simulink model "vllms_4_tap"  (R2021a)
settings: Solver=VariableStepDiscrete  StartTime=0.0  StopTime=4000  MaxStep=1.0  RelTol=1e-3  EnableMultiTasking=on
libraries: dspsrcs4 x2
settings Model: Creator=HP  LastModifiedBy=HP
settings SolverCC: AlgebraicLoopSolver=TrustRegion
settings DataIOCC: ReturnWorkspaceOutputs=off
settings OptimizationCC: LifeSpan=inf
settings DebuggingCC: SFUnexpectedBacktrackingDiag=warning  SFNoUnconditionalDefaultTransitionDiag=warning  SFMachineParentedDataDiag=warning  ArithmeticOperatorsInVariantConditions=warning
settings SFSimCC: SimUseLocalCustomCode=off  CustomCodeUndefinedFunction=UseInterfaceOnly
settings RTWCC: RTWUseLocalCustomCode=off
settings CodeAppCC: StateflowObjectComments=on
settings GRTTargetCC: TargetLangStandard=C89/C90 (ANSI)
settings ConfigComp: CovMetricSettings=dw  CovSaveCumulativeToWorkspaceVar=on  CovSaveSingleToWorkspaceVar=on  CovExternalEMLEnable=off

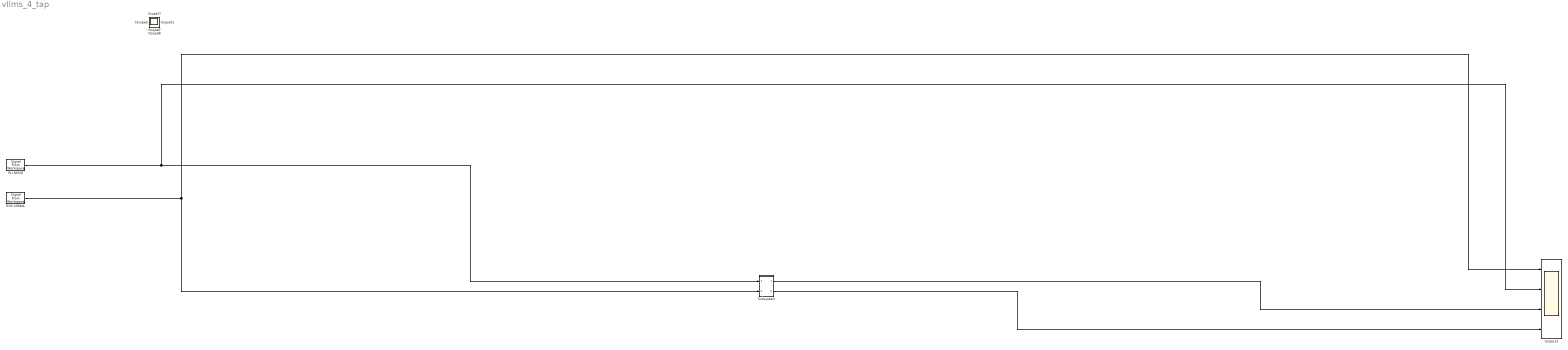
== system vllms_4_tap ==
  ECG SIGNAL : dspsrcs4/Signal From Workspace  X=m1  Ts=1  nsamps=1  OutputAfterFinalValue=Setting to zero  ignoreOrWarnInputAndFrameLengths=off  OutputFrames=off
  PLI NOISE : dspsrcs4/Signal From Workspace  X=x1  Ts=1  nsamps=1  OutputAfterFinalValue=Setting to zero  ignoreOrWarnInputAndFrameLengths=off  OutputFrames=off
  Scope12 : Scope  NumInputPorts=4
  Subsystem : Subsystem
  Scope{,1..11,16..17} (14 alike) : Scope
  wires:
  ECG SIGNAL/1 -> Subsystem/2(In2), Scope12/1
  PLI NOISE/1 -> Subsystem/1(In1), Scope12/2
  Subsystem/1(Out1) -> Scope12/3
  Subsystem/2(Out2) -> Scope12/4

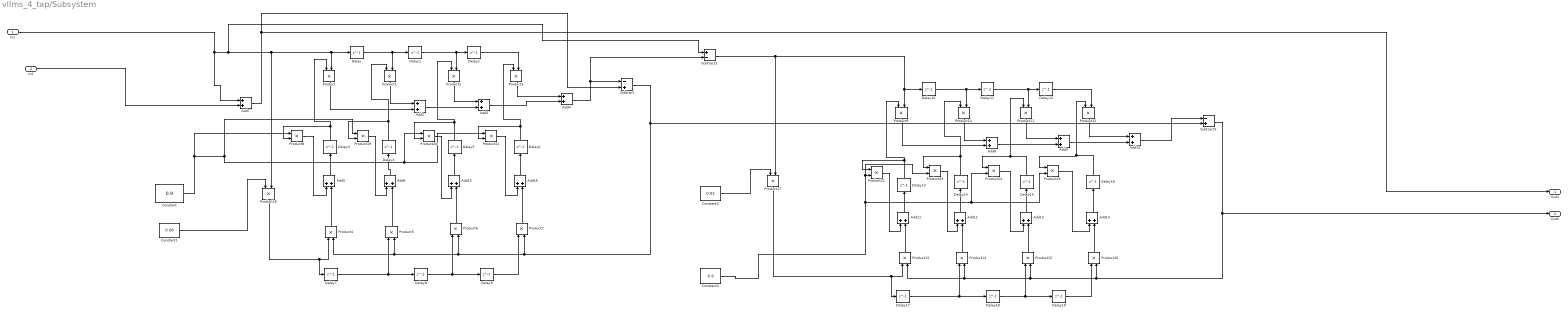
== system vllms_4_tap/Subsystem ==
  In1 : Inport
  In2 : Inport  Port=2
  Add{2..16} (15 alike) : Sum
  Constant : Constant  Value=0.9
  Constant1 : Constant  Value=0.08
  Constant2 : Constant  Value=0.02
  Constant3 : Constant  Value=0.9
  Delay{,1..19} (20 alike) : Delay  DelayLength=1  InitialCondition=0
  Product{,1..25} (26 alike) : Product
  Subtract : Sum  Inputs=-+
  Subtract1 : Sum  Inputs=+-
  Subtract3 : Sum  Inputs=-+
  Out1 : Outport
  Out2 : Outport  Port=2
  wires:
  Subtract1/1 -> Product9/2, Delay10/1, Product17/2
  Delay16/1 -> Product25/1, Product12/1
  Delay11/1 -> Product11/2, Delay12/1
  Product12/1 -> Add10/1
  Subtract3/1 -> Out2/1, Product16/2, Product15/2, Product13/2, Product14/2
  Product11/1 -> Add9/1
  Delay7/1 -> Product5/1, Delay8/1
  In1/1 -> Add7/1, Subtract1/1, Product18/2, Product/2, Delay/1
  Delay9/1 -> Product7/1
  Delay5/1 -> Product20/2, Product2/1
  Delay15/1 -> Product11/1, Product24/1
  Product10/1 -> Add8/1
  Add7/1 -> Subtract/2, Out1/1
  Product14/1 -> Add12/2
  Product24/1 -> Add13/1
  Constant/1 -> Product8/1, Product19/1, Product21/1, Product20/1
  Delay13/1 -> Product22/1, Product9/1
  Add8/1 -> Add9/2
  Add10/1 -> Subtract3/1
  Product20/1 -> Add15/1
  Product13/1 -> Add11/2
  Add2/1 -> Add3/2
  Constant2/1 -> Product17/1
  Delay/1 -> Product1/2, Delay1/1
  Product15/1 -> Add13/2
  Delay3/1 -> Product8/2, Product/1
  Delay14/1 -> Product23/1, Product10/1
  Delay18/1 -> Delay19/1, Product15/1
  Product9/1 -> Add8/2
  Delay19/1 -> Product16/1
  Subtract/1 -> Subtract3/2, Product7/2, Product6/2, Product5/2, Product4/2
  Constant1/1 -> Product18/1
  Add5/1 -> Delay3/1
  Product8/1 -> Add5/1
  Delay17/1 -> Product14/1, Delay18/1
  Product23/1 -> Add12/1
  Product25/1 -> Add14/1
  Constant3/1 -> Product23/2, Product22/2, Product24/2, Product25/2
  Product18/1 -> Product4/1, Delay7/1
  Add12/1 -> Delay14/1
  Add3/1 -> Add4/2
  Add11/1 -> Delay13/1
  Add14/1 -> Delay16/1
  Delay2/1 -> Product3/2
  Add9/1 -> Add10/2
  Add15/1 -> Delay5/1
  Add4/1 -> Subtract1/2, Subtract/1
  Product1/1 -> Add2/1
  Product22/1 -> Add11/1
  Delay6/1 -> Product21/2, Product3/1
  Product17/1 -> Delay17/1, Product13/1
  Product16/1 -> Add14/2
  Delay12/1 -> Product12/2
  Delay10/1 -> Product10/2, Delay11/1
  Add6/1 -> Delay4/1
  Delay4/1 -> Product19/2, Product1/1
  Product21/1 -> Add16/1
  Product5/1 -> Add6/2
  Product6/1 -> Add15/2
  Product19/1 -> Add6/1
  Product7/1 -> Add16/2
  Product4/1 -> Add5/2
  Product/1 -> Add2/2
  Add13/1 -> Delay15/1
  Add16/1 -> Delay6/1
  Delay1/1 -> Product2/2, Delay2/1
  Delay8/1 -> Product6/1, Delay9/1
  Product3/1 -> Add4/1
  Product2/1 -> Add3/1
  In2/1 -> Add7/2
